simulink model "lgg"  (Simulink 7.5)
settings: Solver=ode45  StartTime=0.0  StopTime=5  RelTol=1e-3
values from neighbouring files (symbols this model uses):
  B = [0 ... (first row only)    [system_eq.m]
  J = 0.01    [open_loop.m]    (also in pid_controller.m; system_eq.m)
  K = 0.01    [open_loop.m]    (also in pid_controller.m; system_eq.m)
  L = 0.5    [open_loop.m]    (also in pid_controller.m; system_eq.m)
  R = 1    [open_loop.m]    (also in pid_controller.m; system_eq.m)
settings Model: Creator=B0919120  LastModifiedBy=Victor
settings OptimizationCC: InitFltsAndDblsToZero=on
settings DebuggingCC: StrictBusMsg=Warning

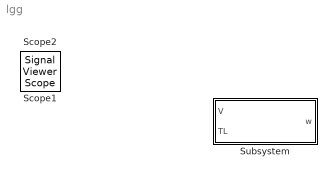
== system lgg ==
  Subsystem : Subsystem
  Scope1 : SignalViewerScope  IOType=viewer  RefreshTime=0.035000
  Scope2 : SignalViewerScope  IOType=viewer  RefreshTime=0.035000

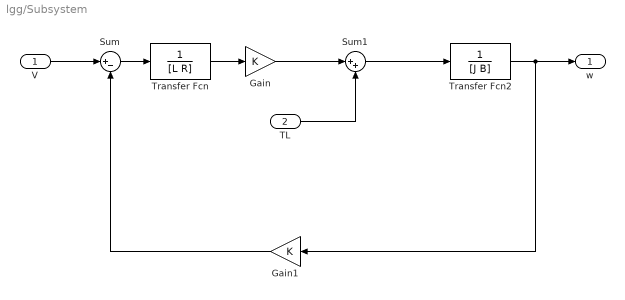
== system lgg/Subsystem ==
  V : Inport  OutDataType=sfix(16)  OutScaling=2^0
  TL : Inport  Port=2  OutDataType=sfix(16)  OutScaling=2^0
  Gain : Gain  Gain=K  ParameterDataType=sfix(16)  ParameterScaling=2^0  OutDataType=sfix(16)  OutScaling=2^0
  Gain1 : Gain  Gain=K  ParameterDataType=sfix(16)  ParameterScaling=2^0  OutDataType=sfix(16)  OutScaling=2^0
  Sum : Sum  Inputs=|+-  OutDataType=sfix(16)  OutScaling=2^0
  Sum1 : Sum  Inputs=|++  OutDataType=sfix(16)  OutScaling=2^0
  Transfer Fcn : TransferFcn  Denominator=[L R]
  Transfer Fcn2 : TransferFcn  Denominator=[J B]
  w : Outport  OutDataType=sfix(16)  OutScaling=2^0
  wires:
  Transfer Fcn2/1 -> w/1, Gain1/1
  Gain1/1 -> Sum/2
  V/1 -> Sum/1
  Sum/1 -> Transfer Fcn/1
  Transfer Fcn/1 -> Gain/1
  Gain/1 -> Sum1/1
  Sum1/1 -> Transfer Fcn2/1
  TL/1 -> Sum1/2
